simulink model "Current_Sensor_PWM_Synchronized"  (R2018a)
settings: Solver=VariableStepAuto  StartTime=0.0  StopTime=10.0  RelTol=1e-3
PreLoadFcn:
  | modelDir = fileparts(get_param(bdroot, 'FileName'));
  | addpath(fullfile(modelDir,'Parameters'));
  | addpath(fullfile(modelDir,'subsystems'));
  | 
  | Parameters_Model
  | Parameters_Simulation
  | Parameters_Estimators
InitFcn:
  | Parameters_Model
  | Parameters_Simulation
  | Parameters_Estimators
undefined symbols (not defined in the file): ADC_Resolution, ADC_Vref, current_sample_end_time_offset, CurrentSense_G, CurrentSense_Rsense, CurrentSense_Voffset, EnableADCquantization, EnableNoise, PWM_Frequency, PWM_Resolution, sensor_sigma2_current_sense
settings Model: Creator=Thomas  LastModifiedBy=Thomas

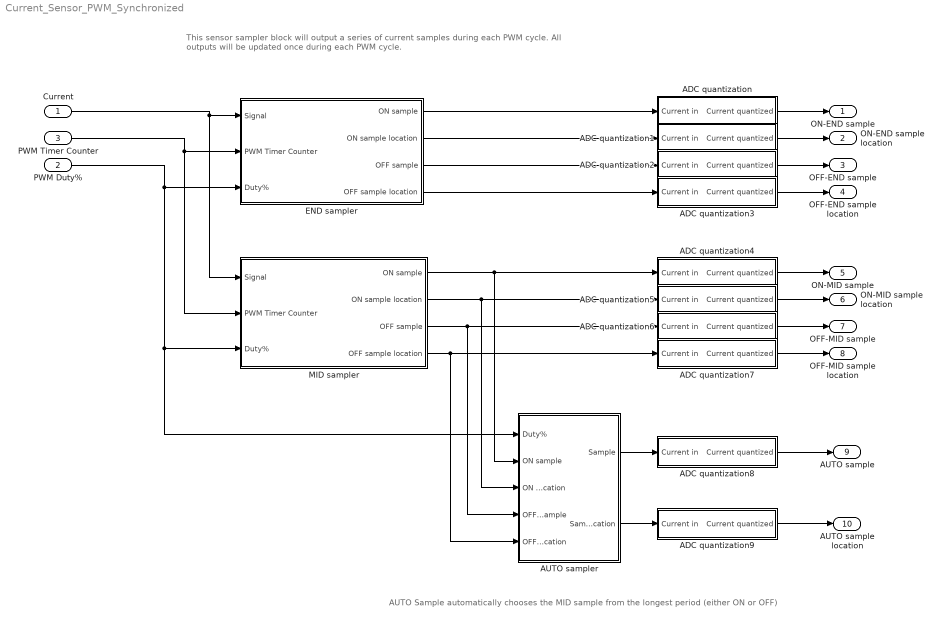
== system Current_Sensor_PWM_Synchronized ==
  note: This sensor sampler block will output a series of current samples during each PWM cycle.
      | All outputs will be updated once during each PWM cycle.
  note: AUTO Sample automatically chooses the MID sample from the longest period (either ON or OFF)
  Current : Inport
  PWM Duty% : Inport  Port=2  OutDataTypeStr=double
  PWM Timer Counter : Inport  Port=3  OutDataTypeStr=uint32  SampleTime=1/(PWM_Resolution*PWM_Frequency)
  ADC quantization : Subsystem
  ADC quantization1 : Subsystem
  ADC quantization2 : Subsystem
  ADC quantization3 : Subsystem
  ADC quantization4 : Subsystem
  ADC quantization5 : Subsystem
  ADC quantization6 : Subsystem
  ADC quantization7 : Subsystem
  ADC quantization8 : Subsystem
  ADC quantization9 : Subsystem
  AUTO sampler : Subsystem
  END sampler : Subsystem
  MID sampler : Subsystem
  ON-END sample : Outport
  ON-END sample location : Outport  Port=2
  OFF-END sample : Outport  Port=3
  OFF-END sample location : Outport  Port=4
  ON-MID sample : Outport  Port=5
  ON-MID sample location : Outport  Port=6
  OFF-MID sample : Outport  Port=7
  OFF-MID sample location : Outport  Port=8
  AUTO sample : Outport  Port=9
  AUTO sample location : Outport  Port=10
  wires:
  AUTO sampler/1(Sample) -> ADC quantization8/1(Current in)
  AUTO sampler/2(Sample location) -> ADC quantization9/1(Current in)
  MID sampler/1(ON sample) -> ADC quantization4/1(Current in), AUTO sampler/2(ON sample)
  MID sampler/2(ON sample location) -> ADC quantization5/1(Current in), AUTO sampler/3(ON sample location)
  MID sampler/3(OFF sample) -> ADC quantization6/1(Current in), AUTO sampler/4(OFF sample)
  MID sampler/4(OFF sample location) -> ADC quantization7/1(Current in), AUTO sampler/5(OFF sample location)
  END sampler/1(ON sample) -> ADC quantization/1(Current in)
  END sampler/2(ON sample location) -> ADC quantization1/1(Current in)
  END sampler/3(OFF sample) -> ADC quantization2/1(Current in)
  END sampler/4(OFF sample location) -> ADC quantization3/1(Current in)
  PWM Duty%/1 -> AUTO sampler/1(Duty%), MID sampler/3(Duty%), END sampler/3(Duty%)
  Current/1 -> MID sampler/1(Signal), END sampler/1(Signal)
  PWM Timer Counter/1 -> MID sampler/2(PWM Timer Counter), END sampler/2(PWM Timer Counter)
  ADC quantization/1(Current quantized) -> ON-END sample/1
  ADC quantization1/1(Current quantized) -> ON-END sample location/1
  ADC quantization2/1(Current quantized) -> OFF-END sample/1
  ADC quantization3/1(Current quantized) -> OFF-END sample location/1
  ADC quantization4/1(Current quantized) -> ON-MID sample/1
  ADC quantization5/1(Current quantized) -> ON-MID sample location/1
  ADC quantization6/1(Current quantized) -> OFF-MID sample/1
  ADC quantization7/1(Current quantized) -> OFF-MID sample location/1
  ADC quantization8/1(Current quantized) -> AUTO sample/1
  ADC quantization9/1(Current quantized) -> AUTO sample location/1

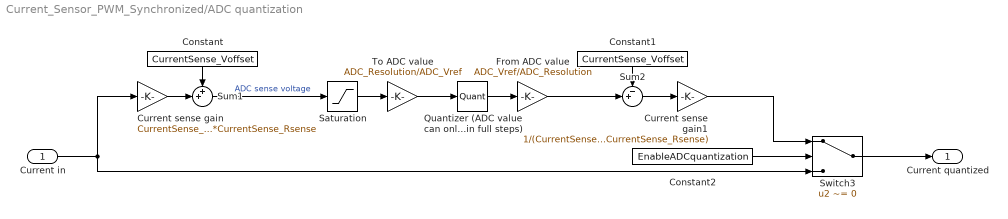
== system Current_Sensor_PWM_Synchronized/ADC quantization ==
  Current in : Inport
  Constant : Constant  Value=CurrentSense_Voffset
  Constant1 : Constant  Value=CurrentSense_Voffset
  Constant2 : Constant  Value=EnableADCquantization
  Current sense gain : Gain  Gain=CurrentSense_G*CurrentSense_Rsense
  Current sense gain1 : Gain  Gain=1/(CurrentSense_G*CurrentSense_Rsense)
  From ADC value : Gain  Gain=ADC_Vref/ADC_Resolution
  Quantizer (ADC value can only be measured in full steps) : Quantizer  QuantizationInterval=1
  Saturation : Saturate  UpperLimit=ADC_Vref  LowerLimit=0
  Sum1 : Sum  Inputs=++|
  Sum2 : Sum  Inputs=-+|
  Switch3 : Switch  Criteria=u2 ~= 0
  To ADC value : Gain  Gain=ADC_Resolution/ADC_Vref
  Current quantized : Outport
  wires:
  Current sense gain/1 -> Sum1/2
  Sum1/1 -> Saturation/1  "ADC sense voltage"
  Sum2/1 -> Current sense gain1/1
  Quantizer (ADC value can only be measured in full steps)/1 -> From ADC value/1
  Constant2/1 -> Switch3/2
  To ADC value/1 -> Quantizer (ADC value can only be measured in full steps)/1
  Constant/1 -> Sum1/1
  Current sense gain1/1 -> Switch3/1
  Switch3/1 -> Current quantized/1
  Constant1/1 -> Sum2/1
  From ADC value/1 -> Sum2/2
  Current in/1 -> Switch3/3, Current sense gain/1
  Saturation/1 -> To ADC value/1

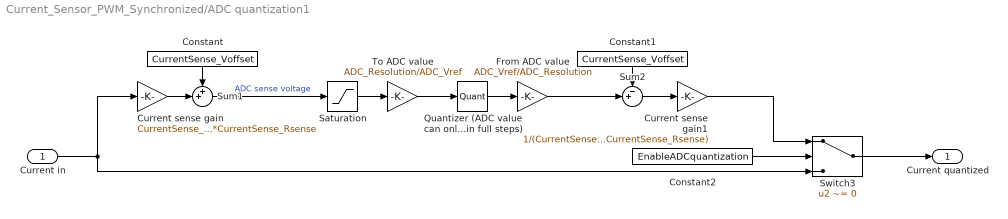
== system Current_Sensor_PWM_Synchronized/ADC quantization1 ==
  Current in : Inport
  Constant : Constant  Value=CurrentSense_Voffset
  Constant1 : Constant  Value=CurrentSense_Voffset
  Constant2 : Constant  Value=EnableADCquantization
  Current sense gain : Gain  Gain=CurrentSense_G*CurrentSense_Rsense
  Current sense gain1 : Gain  Gain=1/(CurrentSense_G*CurrentSense_Rsense)
  From ADC value : Gain  Gain=ADC_Vref/ADC_Resolution
  Quantizer (ADC value can only be measured in full steps) : Quantizer  QuantizationInterval=1
  Saturation : Saturate  UpperLimit=ADC_Vref  LowerLimit=0
  Sum1 : Sum  Inputs=++|
  Sum2 : Sum  Inputs=-+|
  Switch3 : Switch  Criteria=u2 ~= 0
  To ADC value : Gain  Gain=ADC_Resolution/ADC_Vref
  Current quantized : Outport
  wires:
  Current sense gain/1 -> Sum1/2
  Sum1/1 -> Saturation/1  "ADC sense voltage"
  Sum2/1 -> Current sense gain1/1
  Quantizer (ADC value can only be measured in full steps)/1 -> From ADC value/1
  Constant2/1 -> Switch3/2
  To ADC value/1 -> Quantizer (ADC value can only be measured in full steps)/1
  Constant/1 -> Sum1/1
  Current sense gain1/1 -> Switch3/1
  Switch3/1 -> Current quantized/1
  Constant1/1 -> Sum2/1
  From ADC value/1 -> Sum2/2
  Current in/1 -> Switch3/3, Current sense gain/1
  Saturation/1 -> To ADC value/1

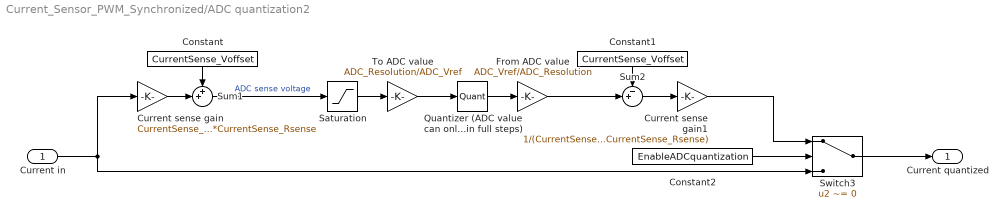
== system Current_Sensor_PWM_Synchronized/ADC quantization2 ==
  Current in : Inport
  Constant : Constant  Value=CurrentSense_Voffset
  Constant1 : Constant  Value=CurrentSense_Voffset
  Constant2 : Constant  Value=EnableADCquantization
  Current sense gain : Gain  Gain=CurrentSense_G*CurrentSense_Rsense
  Current sense gain1 : Gain  Gain=1/(CurrentSense_G*CurrentSense_Rsense)
  From ADC value : Gain  Gain=ADC_Vref/ADC_Resolution
  Quantizer (ADC value can only be measured in full steps) : Quantizer  QuantizationInterval=1
  Saturation : Saturate  UpperLimit=ADC_Vref  LowerLimit=0
  Sum1 : Sum  Inputs=++|
  Sum2 : Sum  Inputs=-+|
  Switch3 : Switch  Criteria=u2 ~= 0
  To ADC value : Gain  Gain=ADC_Resolution/ADC_Vref
  Current quantized : Outport
  wires:
  Current sense gain/1 -> Sum1/2
  Sum1/1 -> Saturation/1  "ADC sense voltage"
  Sum2/1 -> Current sense gain1/1
  Quantizer (ADC value can only be measured in full steps)/1 -> From ADC value/1
  Constant2/1 -> Switch3/2
  To ADC value/1 -> Quantizer (ADC value can only be measured in full steps)/1
  Constant/1 -> Sum1/1
  Current sense gain1/1 -> Switch3/1
  Switch3/1 -> Current quantized/1
  Constant1/1 -> Sum2/1
  From ADC value/1 -> Sum2/2
  Current in/1 -> Switch3/3, Current sense gain/1
  Saturation/1 -> To ADC value/1

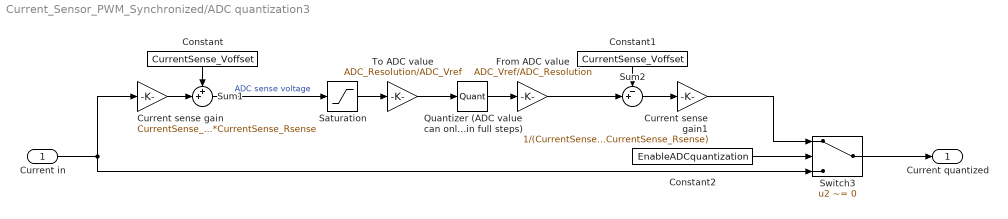
== system Current_Sensor_PWM_Synchronized/ADC quantization3 ==
  Current in : Inport
  Constant : Constant  Value=CurrentSense_Voffset
  Constant1 : Constant  Value=CurrentSense_Voffset
  Constant2 : Constant  Value=EnableADCquantization
  Current sense gain : Gain  Gain=CurrentSense_G*CurrentSense_Rsense
  Current sense gain1 : Gain  Gain=1/(CurrentSense_G*CurrentSense_Rsense)
  From ADC value : Gain  Gain=ADC_Vref/ADC_Resolution
  Quantizer (ADC value can only be measured in full steps) : Quantizer  QuantizationInterval=1
  Saturation : Saturate  UpperLimit=ADC_Vref  LowerLimit=0
  Sum1 : Sum  Inputs=++|
  Sum2 : Sum  Inputs=-+|
  Switch3 : Switch  Criteria=u2 ~= 0
  To ADC value : Gain  Gain=ADC_Resolution/ADC_Vref
  Current quantized : Outport
  wires:
  Current sense gain/1 -> Sum1/2
  Sum1/1 -> Saturation/1  "ADC sense voltage"
  Sum2/1 -> Current sense gain1/1
  Quantizer (ADC value can only be measured in full steps)/1 -> From ADC value/1
  Constant2/1 -> Switch3/2
  To ADC value/1 -> Quantizer (ADC value can only be measured in full steps)/1
  Constant/1 -> Sum1/1
  Current sense gain1/1 -> Switch3/1
  Switch3/1 -> Current quantized/1
  Constant1/1 -> Sum2/1
  From ADC value/1 -> Sum2/2
  Current in/1 -> Switch3/3, Current sense gain/1
  Saturation/1 -> To ADC value/1

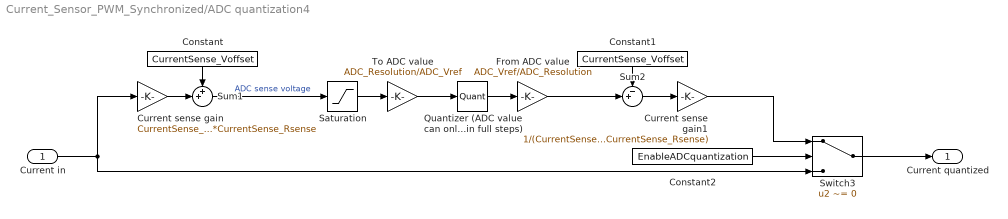
== system Current_Sensor_PWM_Synchronized/ADC quantization4 ==
  Current in : Inport
  Constant : Constant  Value=CurrentSense_Voffset
  Constant1 : Constant  Value=CurrentSense_Voffset
  Constant2 : Constant  Value=EnableADCquantization
  Current sense gain : Gain  Gain=CurrentSense_G*CurrentSense_Rsense
  Current sense gain1 : Gain  Gain=1/(CurrentSense_G*CurrentSense_Rsense)
  From ADC value : Gain  Gain=ADC_Vref/ADC_Resolution
  Quantizer (ADC value can only be measured in full steps) : Quantizer  QuantizationInterval=1
  Saturation : Saturate  UpperLimit=ADC_Vref  LowerLimit=0
  Sum1 : Sum  Inputs=++|
  Sum2 : Sum  Inputs=-+|
  Switch3 : Switch  Criteria=u2 ~= 0
  To ADC value : Gain  Gain=ADC_Resolution/ADC_Vref
  Current quantized : Outport
  wires:
  Current sense gain/1 -> Sum1/2
  Sum1/1 -> Saturation/1  "ADC sense voltage"
  Sum2/1 -> Current sense gain1/1
  Quantizer (ADC value can only be measured in full steps)/1 -> From ADC value/1
  Constant2/1 -> Switch3/2
  To ADC value/1 -> Quantizer (ADC value can only be measured in full steps)/1
  Constant/1 -> Sum1/1
  Current sense gain1/1 -> Switch3/1
  Switch3/1 -> Current quantized/1
  Constant1/1 -> Sum2/1
  From ADC value/1 -> Sum2/2
  Current in/1 -> Switch3/3, Current sense gain/1
  Saturation/1 -> To ADC value/1

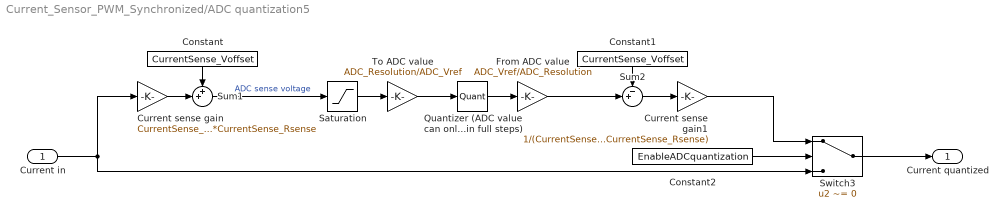
== system Current_Sensor_PWM_Synchronized/ADC quantization5 ==
  Current in : Inport
  Constant : Constant  Value=CurrentSense_Voffset
  Constant1 : Constant  Value=CurrentSense_Voffset
  Constant2 : Constant  Value=EnableADCquantization
  Current sense gain : Gain  Gain=CurrentSense_G*CurrentSense_Rsense
  Current sense gain1 : Gain  Gain=1/(CurrentSense_G*CurrentSense_Rsense)
  From ADC value : Gain  Gain=ADC_Vref/ADC_Resolution
  Quantizer (ADC value can only be measured in full steps) : Quantizer  QuantizationInterval=1
  Saturation : Saturate  UpperLimit=ADC_Vref  LowerLimit=0
  Sum1 : Sum  Inputs=++|
  Sum2 : Sum  Inputs=-+|
  Switch3 : Switch  Criteria=u2 ~= 0
  To ADC value : Gain  Gain=ADC_Resolution/ADC_Vref
  Current quantized : Outport
  wires:
  Current sense gain/1 -> Sum1/2
  Sum1/1 -> Saturation/1  "ADC sense voltage"
  Sum2/1 -> Current sense gain1/1
  Quantizer (ADC value can only be measured in full steps)/1 -> From ADC value/1
  Constant2/1 -> Switch3/2
  To ADC value/1 -> Quantizer (ADC value can only be measured in full steps)/1
  Constant/1 -> Sum1/1
  Current sense gain1/1 -> Switch3/1
  Switch3/1 -> Current quantized/1
  Constant1/1 -> Sum2/1
  From ADC value/1 -> Sum2/2
  Current in/1 -> Switch3/3, Current sense gain/1
  Saturation/1 -> To ADC value/1

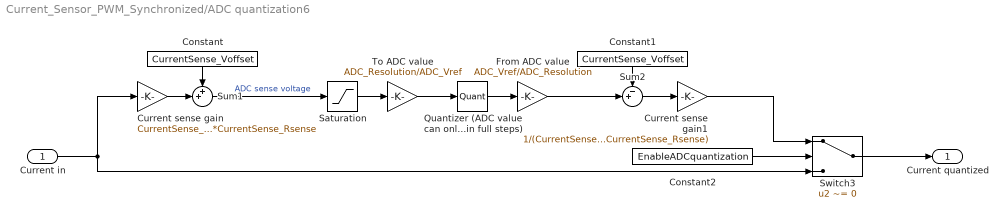
== system Current_Sensor_PWM_Synchronized/ADC quantization6 ==
  Current in : Inport
  Constant : Constant  Value=CurrentSense_Voffset
  Constant1 : Constant  Value=CurrentSense_Voffset
  Constant2 : Constant  Value=EnableADCquantization
  Current sense gain : Gain  Gain=CurrentSense_G*CurrentSense_Rsense
  Current sense gain1 : Gain  Gain=1/(CurrentSense_G*CurrentSense_Rsense)
  From ADC value : Gain  Gain=ADC_Vref/ADC_Resolution
  Quantizer (ADC value can only be measured in full steps) : Quantizer  QuantizationInterval=1
  Saturation : Saturate  UpperLimit=ADC_Vref  LowerLimit=0
  Sum1 : Sum  Inputs=++|
  Sum2 : Sum  Inputs=-+|
  Switch3 : Switch  Criteria=u2 ~= 0
  To ADC value : Gain  Gain=ADC_Resolution/ADC_Vref
  Current quantized : Outport
  wires:
  Current sense gain/1 -> Sum1/2
  Sum1/1 -> Saturation/1  "ADC sense voltage"
  Sum2/1 -> Current sense gain1/1
  Quantizer (ADC value can only be measured in full steps)/1 -> From ADC value/1
  Constant2/1 -> Switch3/2
  To ADC value/1 -> Quantizer (ADC value can only be measured in full steps)/1
  Constant/1 -> Sum1/1
  Current sense gain1/1 -> Switch3/1
  Switch3/1 -> Current quantized/1
  Constant1/1 -> Sum2/1
  From ADC value/1 -> Sum2/2
  Current in/1 -> Switch3/3, Current sense gain/1
  Saturation/1 -> To ADC value/1

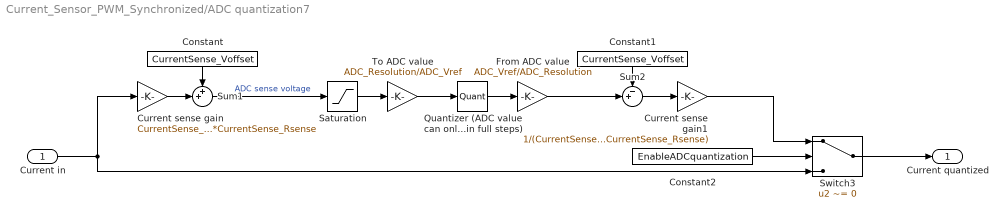
== system Current_Sensor_PWM_Synchronized/ADC quantization7 ==
  Current in : Inport
  Constant : Constant  Value=CurrentSense_Voffset
  Constant1 : Constant  Value=CurrentSense_Voffset
  Constant2 : Constant  Value=EnableADCquantization
  Current sense gain : Gain  Gain=CurrentSense_G*CurrentSense_Rsense
  Current sense gain1 : Gain  Gain=1/(CurrentSense_G*CurrentSense_Rsense)
  From ADC value : Gain  Gain=ADC_Vref/ADC_Resolution
  Quantizer (ADC value can only be measured in full steps) : Quantizer  QuantizationInterval=1
  Saturation : Saturate  UpperLimit=ADC_Vref  LowerLimit=0
  Sum1 : Sum  Inputs=++|
  Sum2 : Sum  Inputs=-+|
  Switch3 : Switch  Criteria=u2 ~= 0
  To ADC value : Gain  Gain=ADC_Resolution/ADC_Vref
  Current quantized : Outport
  wires:
  Current sense gain/1 -> Sum1/2
  Sum1/1 -> Saturation/1  "ADC sense voltage"
  Sum2/1 -> Current sense gain1/1
  Quantizer (ADC value can only be measured in full steps)/1 -> From ADC value/1
  Constant2/1 -> Switch3/2
  To ADC value/1 -> Quantizer (ADC value can only be measured in full steps)/1
  Constant/1 -> Sum1/1
  Current sense gain1/1 -> Switch3/1
  Switch3/1 -> Current quantized/1
  Constant1/1 -> Sum2/1
  From ADC value/1 -> Sum2/2
  Current in/1 -> Switch3/3, Current sense gain/1
  Saturation/1 -> To ADC value/1

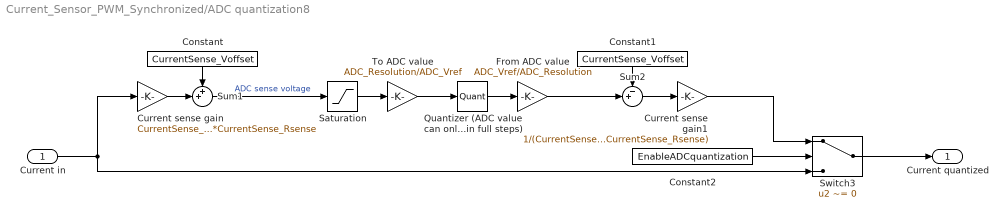
== system Current_Sensor_PWM_Synchronized/ADC quantization8 ==
  Current in : Inport
  Constant : Constant  Value=CurrentSense_Voffset
  Constant1 : Constant  Value=CurrentSense_Voffset
  Constant2 : Constant  Value=EnableADCquantization
  Current sense gain : Gain  Gain=CurrentSense_G*CurrentSense_Rsense
  Current sense gain1 : Gain  Gain=1/(CurrentSense_G*CurrentSense_Rsense)
  From ADC value : Gain  Gain=ADC_Vref/ADC_Resolution
  Quantizer (ADC value can only be measured in full steps) : Quantizer  QuantizationInterval=1
  Saturation : Saturate  UpperLimit=ADC_Vref  LowerLimit=0
  Sum1 : Sum  Inputs=++|
  Sum2 : Sum  Inputs=-+|
  Switch3 : Switch  Criteria=u2 ~= 0
  To ADC value : Gain  Gain=ADC_Resolution/ADC_Vref
  Current quantized : Outport
  wires:
  Current sense gain/1 -> Sum1/2
  Sum1/1 -> Saturation/1  "ADC sense voltage"
  Sum2/1 -> Current sense gain1/1
  Quantizer (ADC value can only be measured in full steps)/1 -> From ADC value/1
  Constant2/1 -> Switch3/2
  To ADC value/1 -> Quantizer (ADC value can only be measured in full steps)/1
  Constant/1 -> Sum1/1
  Current sense gain1/1 -> Switch3/1
  Switch3/1 -> Current quantized/1
  Constant1/1 -> Sum2/1
  From ADC value/1 -> Sum2/2
  Current in/1 -> Switch3/3, Current sense gain/1
  Saturation/1 -> To ADC value/1

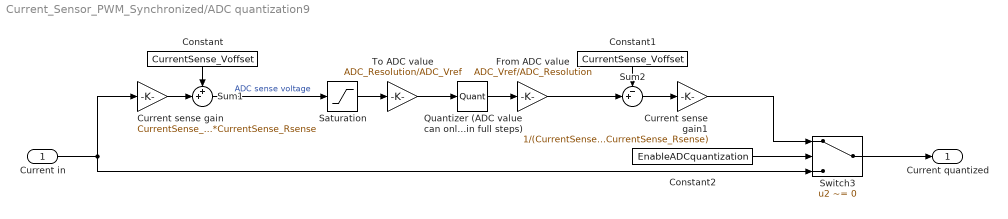
== system Current_Sensor_PWM_Synchronized/ADC quantization9 ==
  Current in : Inport
  Constant : Constant  Value=CurrentSense_Voffset
  Constant1 : Constant  Value=CurrentSense_Voffset
  Constant2 : Constant  Value=EnableADCquantization
  Current sense gain : Gain  Gain=CurrentSense_G*CurrentSense_Rsense
  Current sense gain1 : Gain  Gain=1/(CurrentSense_G*CurrentSense_Rsense)
  From ADC value : Gain  Gain=ADC_Vref/ADC_Resolution
  Quantizer (ADC value can only be measured in full steps) : Quantizer  QuantizationInterval=1
  Saturation : Saturate  UpperLimit=ADC_Vref  LowerLimit=0
  Sum1 : Sum  Inputs=++|
  Sum2 : Sum  Inputs=-+|
  Switch3 : Switch  Criteria=u2 ~= 0
  To ADC value : Gain  Gain=ADC_Resolution/ADC_Vref
  Current quantized : Outport
  wires:
  Current sense gain/1 -> Sum1/2
  Sum1/1 -> Saturation/1  "ADC sense voltage"
  Sum2/1 -> Current sense gain1/1
  Quantizer (ADC value can only be measured in full steps)/1 -> From ADC value/1
  Constant2/1 -> Switch3/2
  To ADC value/1 -> Quantizer (ADC value can only be measured in full steps)/1
  Constant/1 -> Sum1/1
  Current sense gain1/1 -> Switch3/1
  Switch3/1 -> Current quantized/1
  Constant1/1 -> Sum2/1
  From ADC value/1 -> Sum2/2
  Current in/1 -> Switch3/3, Current sense gain/1
  Saturation/1 -> To ADC value/1

== system Current_Sensor_PWM_Synchronized/AUTO sampler ==
  Duty% : Inport  OutDataTypeStr=double
  ON sample : Inport  Port=2
  ON sample location : Inport  Port=3
  OFF sample : Inport  Port=4
  OFF sample location : Inport  Port=5
  Switch : Switch  Threshold=0.5
  Switch1 : Switch  Threshold=0.5
  Sample : Outport
  Sample location : Outport  Port=2
  wires:
  Duty%/1 -> Switch1/2, Switch/2
  ON sample/1 -> Switch/1
  OFF sample/1 -> Switch/3
  Switch/1 -> Sample/1
  OFF sample location/1 -> Switch1/3
  ON sample location/1 -> Switch1/1
  Switch1/1 -> Sample location/1

== system Current_Sensor_PWM_Synchronized/END sampler ==
  Signal : Inport
  PWM Timer Counter : Inport  Port=2
  Duty% : Inport  Port=3  OutDataTypeStr=double
  Abs : Abs
  OFF-end sampler : Subsystem
  ON-end sampler : Subsystem
  ON sample : Outport
  ON sample location : Outport  Port=2
  OFF sample : Outport  Port=3
  OFF sample location : Outport  Port=4
  wires:
  Signal/1 -> OFF-end sampler/1(Signal), ON-end sampler/1(Signal)
  ON-end sampler/1(Sample) -> ON sample/1
  Duty%/1 -> Abs/1
  OFF-end sampler/1(Sample) -> OFF sample/1
  ON-end sampler/2(Sample location) -> ON sample location/1
  OFF-end sampler/2(Sample location) -> OFF sample location/1
  PWM Timer Counter/1 -> ON-end sampler/2(PWM Timer Counter), OFF-end sampler/2(PWM Timer Counter)
  Abs/1 -> ON-end sampler/3(Duty%)

== system Current_Sensor_PWM_Synchronized/MID sampler ==
  Signal : Inport
  PWM Timer Counter : Inport  Port=2
  Duty% : Inport  Port=3  OutDataTypeStr=double
  Abs : Abs
  OFF-mid sampler : Subsystem
  ON-mid sampler : Subsystem
  ON sample : Outport
  ON sample location : Outport  Port=2
  OFF sample : Outport  Port=3
  OFF sample location : Outport  Port=4
  wires:
  Signal/1 -> ON-mid sampler/1(Signal), OFF-mid sampler/1(Signal)
  ON-mid sampler/1(Sample) -> ON sample/1
  Duty%/1 -> Abs/1
  OFF-mid sampler/1(Sample) -> OFF sample/1
  ON-mid sampler/2(Sample location) -> ON sample location/1
  OFF-mid sampler/2(Sample location) -> OFF sample location/1
  PWM Timer Counter/1 -> ON-mid sampler/2(PWM Timer Counter), OFF-mid sampler/2(PWM Timer Counter)
  Abs/1 -> ON-mid sampler/3(Duty%), OFF-mid sampler/3(Duty%)

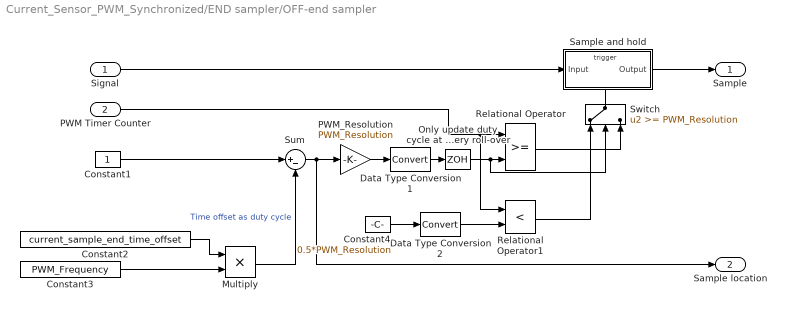
== system Current_Sensor_PWM_Synchronized/END sampler/OFF-end sampler ==
  Signal : Inport
  PWM Timer Counter : Inport  Port=2
  Constant1 : Constant
  Constant2 : Constant  Value=current_sample_end_time_offset
  Constant3 : Constant  Value=PWM_Frequency
  Constant4 : Constant  Value=0.5*PWM_Resolution
  Data Type Conversion1 : DataTypeConversion  RndMeth=Round
  Data Type Conversion2 : DataTypeConversion  RndMeth=Round
  Multiply : Product
  Only update duty cycle at every roll-over : ZeroOrderHold  SampleTime=1/PWM_Frequency
  PWM_Resolution : Gain  Gain=PWM_Resolution
  Relational Operator : RelationalOperator  OutDataTypeStr=boolean  RndMeth=Simplest
  Relational Operator1 : RelationalOperator  Operator=<  OutDataTypeStr=boolean  RndMeth=Simplest
  Sample and hold : Subsystem
  Sum : Sum  Inputs=|+-
  Switch : Switch  Threshold=PWM_Resolution
  Sample : Outport
  Sample location : Outport  Port=2
  wires:
  Only update duty cycle at every roll-over/1 -> Switch/2, Relational Operator/2
  PWM Timer Counter/1 -> Relational Operator/1, Relational Operator1/1
  Signal/1 -> Sample and hold/1(Input)
  Data Type Conversion1/1 -> Only update duty cycle at every roll-over/1
  Sum/1 -> Sample location/1, PWM_Resolution/1
  Sample and hold/1(Output) -> Sample/1
  Constant1/1 -> Sum/1
  PWM_Resolution/1 -> Data Type Conversion1/1
  Constant2/1 -> Multiply/1
  Multiply/1 -> Sum/2  "Time offset as duty cycle"
  Constant3/1 -> Multiply/2
  Constant4/1 -> Data Type Conversion2/1
  Data Type Conversion2/1 -> Relational Operator1/2
  Relational Operator1/1 -> Switch/1
  Switch/1 -> Sample and hold/Trigger
  Relational Operator/1 -> Switch/3

== system Current_Sensor_PWM_Synchronized/END sampler/ON-end sampler ==
  note: Only update duty cycle at every roll-over
  Signal : Inport
  PWM Timer Counter : Inport  Port=2
  Duty% : Inport  Port=3  OutDataTypeStr=double
  Constant1 : Constant  Value=current_sample_end_time_offset
  Constant2 : Constant  Value=PWM_Frequency
  Data Type Conversion1 : DataTypeConversion  RndMeth=Round
  Multiply : Product
  PWM_Resolution : Gain  Gain=PWM_Resolution
  Relational Operator : RelationalOperator  Operator=<  OutDataTypeStr=boolean  RndMeth=Simplest
  Sample and hold with noise : Subsystem
  Sum : Sum  Inputs=|+-
  Zero-Order Hold : ZeroOrderHold  SampleTime=1/PWM_Frequency
  Sample : Outport
  Sample location : Outport  Port=2
  wires:
  Relational Operator/1 -> Sample and hold with noise/Trigger
  Zero-Order Hold/1 -> Relational Operator/2
  PWM Timer Counter/1 -> Relational Operator/1
  Signal/1 -> Sample and hold with noise/1(Input)
  Data Type Conversion1/1 -> Zero-Order Hold/1
  Sum/1 -> PWM_Resolution/1, Sample location/1
  Sample and hold with noise/1(Output) -> Sample/1
  Duty%/1 -> Sum/1
  PWM_Resolution/1 -> Data Type Conversion1/1
  Constant1/1 -> Multiply/1
  Constant2/1 -> Multiply/2
  Multiply/1 -> Sum/2  "Time offset as duty cycle"

== system Current_Sensor_PWM_Synchronized/MID sampler/OFF-mid sampler ==
  note: Only update duty cycle at every roll-over
  note: Sample in the middle of OFF-period @ 1-(0.5*(1-duty)) = 0.5+0.5*duty
  Signal : Inport
  PWM Timer Counter : Inport  Port=2
  Duty% : Inport  Port=3  OutDataTypeStr=double
  Constant : Constant
  Data Type Conversion1 : DataTypeConversion  RndMeth=Round
  Gain : Gain  Gain=0.5
  PWM_Resolution : Gain  Gain=PWM_Resolution
  Relational Operator : RelationalOperator  Operator=<  OutDataTypeStr=boolean  RndMeth=Simplest
  Sample and hold : Subsystem
  Sum : Sum  Inputs=-+|
  Sum1 : Sum  Inputs=|-+
  Zero-Order Hold : ZeroOrderHold  SampleTime=1/PWM_Frequency
  Sample : Outport
  Sample location : Outport  Port=2
  wires:
  Relational Operator/1 -> Sample and hold/Trigger
  Zero-Order Hold/1 -> Relational Operator/2
  PWM Timer Counter/1 -> Relational Operator/1
  Signal/1 -> Sample and hold/1(Input)
  Data Type Conversion1/1 -> Zero-Order Hold/1
  Sum1/1 -> PWM_Resolution/1, Sample location/1
  Sample and hold/1(Output) -> Sample/1
  PWM_Resolution/1 -> Data Type Conversion1/1
  Duty%/1 -> Sum/1
  Sum/1 -> Gain/1
  Constant/1 -> Sum1/2, Sum/2
  Gain/1 -> Sum1/1

== system Current_Sensor_PWM_Synchronized/MID sampler/ON-mid sampler ==
  note: Sample in the middle of ON-period @ 0.5*duty
  note: Only update duty cycle at every roll-over
  Signal : Inport
  PWM Timer Counter : Inport  Port=2
  Duty% : Inport  Port=3  OutDataTypeStr=double
  Data Type Conversion1 : DataTypeConversion  RndMeth=Round
  Gain : Gain  Gain=0.5
  PWM_Resolution : Gain  Gain=PWM_Resolution
  Relational Operator : RelationalOperator  Operator=<  OutDataTypeStr=boolean  RndMeth=Simplest
  Sample and hold : Subsystem
  Zero-Order Hold : ZeroOrderHold  SampleTime=1/PWM_Frequency
  Sample : Outport
  Sample location : Outport  Port=2
  wires:
  Relational Operator/1 -> Sample and hold/Trigger
  Zero-Order Hold/1 -> Relational Operator/2
  PWM Timer Counter/1 -> Relational Operator/1
  Signal/1 -> Sample and hold/1(Input)
  Data Type Conversion1/1 -> Zero-Order Hold/1
  Gain/1 -> PWM_Resolution/1, Sample location/1
  Sample and hold/1(Output) -> Sample/1
  Duty%/1 -> Gain/1
  PWM_Resolution/1 -> Data Type Conversion1/1

== system Current_Sensor_PWM_Synchronized/END sampler/OFF-end sampler/Sample and hold ==
  Input : Inport
  Trigger : TriggerPort  VariantControl=Variant  PortDimensions=1
  Noise : RandomNumber  Variance=sensor_sigma2_current_sense  Seed=3
  Noise switch : Subsystem
  Sum2 : Sum  Inputs=++|
  Output : Outport
  wires:
  Noise/1 -> Noise switch/1(in)
  Input/1 -> Sum2/2
  Noise switch/1(out) -> Sum2/1
  Sum2/1 -> Output/1

== system Current_Sensor_PWM_Synchronized/END sampler/ON-end sampler/Sample and hold with noise ==
  Input : Inport
  Trigger : TriggerPort  TriggerType=falling  VariantControl=Variant  PortDimensions=1
  Noise : RandomNumber  Variance=sensor_sigma2_current_sense  Seed=2
  Noise switch : Subsystem
  Sum2 : Sum  Inputs=++|
  Output : Outport
  wires:
  Noise/1 -> Noise switch/1(in)
  Input/1 -> Sum2/2
  Noise switch/1(out) -> Sum2/1
  Sum2/1 -> Output/1

== system Current_Sensor_PWM_Synchronized/MID sampler/OFF-mid sampler/Sample and hold ==
  Input : Inport
  Trigger : TriggerPort  TriggerType=falling  VariantControl=Variant  PortDimensions=1
  Noise : RandomNumber  Variance=sensor_sigma2_current_sense  Seed=5
  Noise switch : Subsystem
  Sum2 : Sum  Inputs=++|
  Output : Outport
  wires:
  Sum2/1 -> Output/1
  Input/1 -> Sum2/2
  Noise/1 -> Noise switch/1(in)
  Noise switch/1(out) -> Sum2/1

== system Current_Sensor_PWM_Synchronized/MID sampler/ON-mid sampler/Sample and hold ==
  Input : Inport
  Trigger : TriggerPort  TriggerType=falling  VariantControl=Variant  PortDimensions=1
  Noise : RandomNumber  Variance=sensor_sigma2_current_sense  Seed=4
  Noise switch : Subsystem
  Sum2 : Sum  Inputs=++|
  Output : Outport
  wires:
  Sum2/1 -> Output/1
  Input/1 -> Sum2/2
  Noise/1 -> Noise switch/1(in)
  Noise switch/1(out) -> Sum2/1

== system Current_Sensor_PWM_Synchronized/END sampler/OFF-end sampler/Sample and hold/Noise switch ==
  in : Inport
  Enable noise : Constant  Value=EnableNoise
  No noise : Constant  Value=0
  Switch : Switch  Criteria=u2 > Threshold
  out : Outport
  wires:
  No noise/1 -> Switch/3
  Switch/1 -> out/1
  Enable noise/1 -> Switch/2
  in/1 -> Switch/1

== system Current_Sensor_PWM_Synchronized/END sampler/ON-end sampler/Sample and hold with noise/Noise switch ==
  in : Inport
  Enable noise : Constant  Value=EnableNoise
  No noise : Constant  Value=0
  Switch : Switch  Criteria=u2 > Threshold
  out : Outport
  wires:
  No noise/1 -> Switch/3
  Switch/1 -> out/1
  Enable noise/1 -> Switch/2
  in/1 -> Switch/1

== system Current_Sensor_PWM_Synchronized/MID sampler/OFF-mid sampler/Sample and hold/Noise switch ==
  in : Inport
  Enable noise : Constant  Value=EnableNoise
  No noise : Constant  Value=0
  Switch : Switch  Criteria=u2 > Threshold
  out : Outport
  wires:
  No noise/1 -> Switch/3
  Switch/1 -> out/1
  Enable noise/1 -> Switch/2
  in/1 -> Switch/1

== system Current_Sensor_PWM_Synchronized/MID sampler/ON-mid sampler/Sample and hold/Noise switch ==
  in : Inport
  Enable noise : Constant  Value=EnableNoise
  No noise : Constant  Value=0
  Switch : Switch  Criteria=u2 > Threshold
  out : Outport
  wires:
  No noise/1 -> Switch/3
  Switch/1 -> out/1
  Enable noise/1 -> Switch/2
  in/1 -> Switch/1
